simulink model "pendule_inv_capteur_etu"  (R2021a)
settings: Solver=VariableStepAuto  StartTime=0.0  StopTime=10.0  RelTol=1e-3
values from neighbouring files (symbols this model uses):
  g = 9.81    [simu_pendule_inv_capteur_etu.m]    (also in simu_pendule_inv_echant_etu.m; simu_pendule_inv_etu.m)
  K = [10 1]    [simu_pendule_inv_capteur_etu.m]    (also in simu_pendule_inv_echant_etu.m = [30 10]; simu_pendule_inv_etu.m = [30 10])
  l = 10    [simu_pendule_inv_capteur_etu.m]    (also in simu_pendule_inv_echant_etu.m; simu_pendule_inv_etu.m)
  ue = 0    [simu_pendule_inv_capteur_etu.m]    (also in simu_pendule_inv_echant_etu.m; simu_pendule_inv_etu.m)
  x0 = [pi/20 0]'    [simu_pendule_inv_capteur_etu.m]    (also in simu_pendule_inv_echant_etu.m; simu_pendule_inv_etu.m = [pi/10 0]')
  xe = [0 0]'    [simu_pendule_inv_capteur_etu.m]    (also in simu_pendule_inv_echant_etu.m; simu_pendule_inv_etu.m)
settings Model: Creator=tbonetto  LastModifiedBy=tbonetto

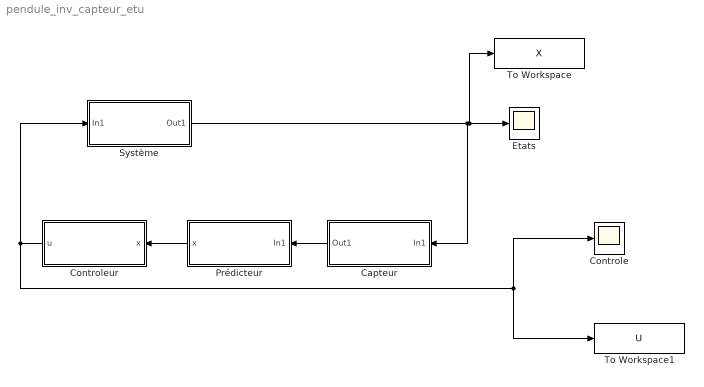
== system pendule_inv_capteur_etu ==
  Capteur : Subsystem
  Controle : Scope
  Controleur : Subsystem
  Etats : Scope
  Prédicteur : Subsystem
  Système : Subsystem
  To Workspace : ToWorkspace  VariableName=X  SaveFormat=Timeseries  SampleTime=-1
  To Workspace1 : ToWorkspace  VariableName=U  SaveFormat=Timeseries  SampleTime=-1
  wires:
  Système/1(Out1) -> Capteur/1(In1), To Workspace/1, Etats/1
  Controleur/1(u) -> Système/1(In1), To Workspace1/1, Controle/1
  Prédicteur/1(x) -> Controleur/1(x)
  Capteur/1(Out1) -> Prédicteur/1(In1)

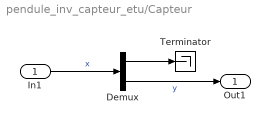
== system pendule_inv_capteur_etu/Capteur ==
  In1 : Inport
  Demux : Demux  Outputs=2
  Terminator : Terminator
  Out1 : Outport
  wires:
  In1/1 -> Demux/1  "x"
  Demux/1 -> Terminator/1
  Demux/2 -> Out1/1  "y"

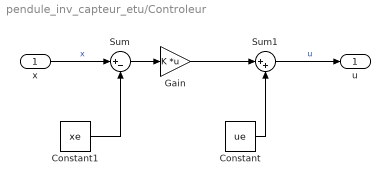
== system pendule_inv_capteur_etu/Controleur ==
  x : Inport
  Constant : Constant  Value=ue
  Constant1 : Constant  Value=xe
  Gain : Gain  Gain=K  Multiplication=Matrix(K*u)
  Sum : Sum  Inputs=|+-
  Sum1 : Sum  Inputs=|++
  u : Outport
  wires:
  Constant/1 -> Sum1/2
  x/1 -> Sum/1  "x"
  Constant1/1 -> Sum/2
  Sum/1 -> Gain/1
  Gain/1 -> Sum1/1
  Sum1/1 -> u/1  "u"

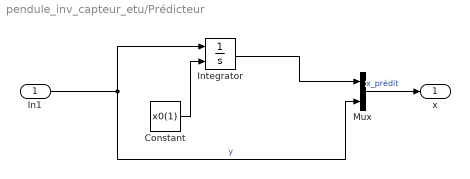
== system pendule_inv_capteur_etu/Prédicteur ==
  In1 : Inport
  Constant : Constant  Value=x0(1)
  Integrator : Integrator  InitialConditionSource=external
  Mux : Mux  Inputs=2
  x : Outport
  wires:
  Mux/1 -> x/1  "x_prédit"
  Integrator/1 -> Mux/1
  In1/1 -> Integrator/1, Mux/2  "y"
  Constant/1 -> Integrator/2

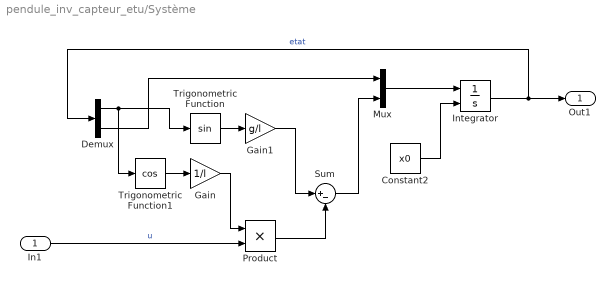
== system pendule_inv_capteur_etu/Système ==
  In1 : Inport
  Constant2 : Constant  Value=x0
  Demux : Demux  Outputs=2
  Gain : Gain  Gain=1/l
  Gain1 : Gain  Gain=g/l
  Integrator : Integrator  InitialConditionSource=external
  Mux : Mux  Inputs=2
  Product : Product
  Sum : Sum  Inputs=|+-
  Trigonometric Function : Trigonometry
  Trigonometric Function1 : Trigonometry  Operator=cos
  Out1 : Outport
  wires:
  Integrator/1 -> Demux/1, Out1/1  "etat"
  Constant2/1 -> Integrator/2
  Mux/1 -> Integrator/1
  Demux/2 -> Mux/1
  Demux/1 -> Trigonometric Function1/1, Trigonometric Function/1
  Trigonometric Function1/1 -> Gain/1
  In1/1 -> Product/2  "u"
  Gain/1 -> Product/1
  Trigonometric Function/1 -> Gain1/1
  Gain1/1 -> Sum/1
  Product/1 -> Sum/2
  Sum/1 -> Mux/2
